simulink model "JT_60SA_scheme_japanese_sensors_isoflux_test_XSC"  (R2018a)
settings: Solver=ode45  StartTime=startTime-neg_time  StopTime=stopTime  FixedStep=5e-3  RelTol=1e-5
StartFcn:
  | coder.extrinsic('system');
  |  system('./run.csh')
  | 
  | 
  | 
  | disp('Called of the 1st part of the run.csh')
StopFcn:
  | close all
  | %figure
  | %run('../../JT-60SA simulation scheme/testPlot.m')
values from neighbouring files (symbols this model uses):
  A_contr = A    [JT60_CD_Invessel_simulator.m]    (also in JT_60SA_SOF18d66_japs_sensors_isoflux_simulator.m; JT_60SA_simulator_VS_SOF18d66_japs_sensors_isoflux_sqzd.m; getABCD (1).m = real(A_contr); getABCD.m = real(A_contr))
  B_contr = [B(:,[1:12 end]) A_contr*E]    [JT60_CD_Invessel_simulator.m]    (also in JT_60SA_SOF18d66_japs_sensors_isoflux_simulator.m; JT_60SA_simulator_VS_SOF18d66_japs_sensors_isoflux_sqzd.m; getABCD (1).m = [B_contr zeros(size(B_contr, 1), 2)]; getABCD.m = [B_contr, E([indexVD, indexEddy], :), Edot([indexVD, indexEd)
  C_contr = LinearModel.C(outputIdx,:)    [JT60_CD_Invessel_simulator.m]    (also in JT_60SA_SOF18d66_japs_sensors_isoflux_simulator.m; JT_60SA_simulator_VS_SOF18d66_japs_sensors_isoflux_sqzd.m; getABCD (1).m = [C1 C2] * T1; getABCD.m = [C1 C2] * T1)
  C_XSC_full = [C_PsiD; C_RxZx]    [XSC_isoflux_FBC.m]
  CSsat = [1 1.0 1.0 1] * 1e3    [JT60_CD_Invessel_simulator.m]    (also in JT_60SA_SOF18d66_japs_sensors_isoflux_simulator.m = [1 1.3 1.3 1] * 1e3; JT_60SA_simulator_VS_SOF18d66_japs_sensors_isoflux_sqzd.m = [1 1.3 1.3 1] * 1e3)
  D_contr = [LinearModel.D(outputIdx,[1:12 end]) LinearModel.F(outputIdx,:)+C_contr*E]    [JT60_CD_Invessel_simulator.m]    (also in JT_60SA_SOF18d66_japs_sensors_isoflux_simulator.m; JT_60SA_simulator_VS_SOF18d66_japs_sensors_isoflux_sqzd.m; getABCD (1).m = [D_contr zeros(size(C_contr, 1), 2)]; getABCD.m = [D_contr, D3])
  EFsat = [1 1.0 1.0 1.0 1.0 1] * 1e3    [JT60_CD_Invessel_simulator.m]    (also in JT_60SA_SOF18d66_japs_sensors_isoflux_simulator.m = [1 .97 .97 .97 .97 1] * 1e3; JT_60SA_simulator_VS_SOF18d66_japs_sensors_isoflux_sqzd.m = [1 .97 .97 .97 .97 1] * 1e3)
  equilDist = LinearModel.YEquil(LinearModel.DisturbancesInfo.OutputPosition)    [JT60_CD_Invessel_simulator.m]    (also in JT_60SA_SOF18d66_japs_sensors_isoflux_simulator.m; JT_60SA_simulator_VS_SOF18d66_japs_sensors_isoflux_sqzd.m)
  equilOutputs = LinearModel.YEquil(outputIdx)    [JT60_CD_Invessel_simulator.m]    (also in JT_60SA_SOF18d66_japs_sensors_isoflux_simulator.m; JT_60SA_simulator_VS_SOF18d66_japs_sensors_isoflux_sqzd.m)
  equilRxZx = LinearModel.YEquil(xIdx)    [JT60_CD_Invessel_simulator.m]    (also in JT_60SA_SOF18d66_japs_sensors_isoflux_simulator.m; JT_60SA_simulator_VS_SOF18d66_japs_sensors_isoflux_sqzd.m)
  equilVolts = zeros(11,1)    [JT60_CD_Invessel_simulator.m]    (also in JT_60SA_SOF18d66_japs_sensors_isoflux_simulator.m = zeros(13,1); JT_60SA_simulator_VS_SOF18d66_japs_sensors_isoflux_sqzd.m = zeros(13,1))
  eqXSC = [eqPsiCntr(2:end)-eqPsiX; eqRxZx]    [XSC_isoflux_FBC.m]
  I_sat_lower = [-3 -3 -3 -3 -3 -3 -3 -3 -3 -3]*1e4    [JT60_CD_Invessel_simulator.m]    (also in JT_60SA_SOF18d66_japs_sensors_isoflux_simulator.m = [-2 -2 -2 -2 -2 -2 -2 -2 -2 -2]*1e4; JT_60SA_simulator_VS_SOF18d66_japs_sensors_isoflux_sqzd.m = [-2 -2 -2 -2 -2 -2 -2 -2 -2 -2]*1e4)
  I_sat_upper = [3 3 3 3 3 3 3 3 3 3]*1e4    [JT60_CD_Invessel_simulator.m]    (also in JT_60SA_SOF18d66_japs_sensors_isoflux_simulator.m = [2 2 2 2 1 1 2 2 1 1]*1e4; JT_60SA_simulator_VS_SOF18d66_japs_sensors_isoflux_sqzd.m = [2 2 2 2 1 1 2 2 1 1]*1e4)
  kIp = kIp/norm(kIp)    [JT60_CD_Invessel_simulator.m]    (also in JT_60SA_SOF18d66_japs_sensors_isoflux_simulator.m; JT_60SA_simulator_VS_SOF18d66_japs_sensors_isoflux_sqzd.m)
  nOfFluxCntrl = nOfFluxCntrl +1    [JT60_CD_Invessel_simulator.m]    (also in JT_60SA_SOF18d66_japs_sensors_isoflux_simulator.m; JT_60SA_simulator_VS_SOF18d66_japs_sensors_isoflux_sqzd.m; MainConfigurator.m = 19)
  nOfFluxSens = 34    [JT60_CD_Invessel_simulator.m]    (also in JT_60SA_SOF18d66_japs_sensors_isoflux_simulator.m; JT_60SA_simulator_VS_SOF18d66_japs_sensors_isoflux_sqzd.m)
  nOfGaps = 85    [JT60_CD_Invessel_simulator.m]    (also in JT_60SA_SOF18d66_japs_sensors_isoflux_simulator.m; JT_60SA_simulator_VS_SOF18d66_japs_sensors_isoflux_sqzd.m)
  nOfMagneticSens = 45    [JT60_CD_Invessel_simulator.m]    (also in JT_60SA_SOF18d66_japs_sensors_isoflux_simulator.m; JT_60SA_simulator_VS_SOF18d66_japs_sensors_isoflux_sqzd.m)
  nOfStrikes = 8    [JT60_CD_Invessel_simulator.m]    (also in JT_60SA_SOF18d66_japs_sensors_isoflux_simulator.m; JT_60SA_simulator_VS_SOF18d66_japs_sensors_isoflux_sqzd.m)
  nXSC = size(C_XSC,1)    [XSC_isoflux_FBC.m]
  PSdelay = 1.5e-3    (= 0.0015)    [JT60_CD_Invessel_simulator.m]    (also in JT_60SA_SOF18d66_japs_sensors_isoflux_simulator.m; JT_60SA_simulator_VS_SOF18d66_japs_sensors_isoflux_sqzd.m)
  PSmodel = tf([1],[PStau 1]) * eye(nPF)    [JT60_CD_Invessel_simulator.m]    (also in JT_60SA_SOF18d66_japs_sensors_isoflux_simulator.m; JT_60SA_simulator_VS_SOF18d66_japs_sensors_isoflux_sqzd.m)
  r_cntrl_gap_eq = r_gap+initialGaps.*cosd(theta_cntrl_gap)    [JT60_CD_Invessel_simulator.m]    (also in JT_60SA_SOF18d66_japs_sensors_isoflux_simulator.m; JT_60SA_simulator_VS_SOF18d66_japs_sensors_isoflux_sqzd.m)
  vLoop = LinearModel.R(end,end)*Ip0    [JT60_CD_Invessel_simulator.m]    (also in JT_60SA_SOF18d66_japs_sensors_isoflux_simulator.m; JT_60SA_simulator_VS_SOF18d66_japs_sensors_isoflux_sqzd.m)
  xi0 = zeros(1, size(A_contr, 1))    [JT60_CD_Invessel_simulator.m]    (also in JT_60SA_SOF18d66_japs_sensors_isoflux_simulator.m; JT_60SA_simulator_VS_SOF18d66_japs_sensors_isoflux_sqzd.m)
  XSC_matrix = XSC_matrix(:, 1:end-1)    [XSC_3rd_try.m]    (also in XSC_SOF.mat = [-142.52465816 14.2057775457 0.338794355553 374.122305988 13; XSC_SOF_flux.mat = [-263113.154477 -155619.089697 161941.063761 -300901.385526 ; XSC_isoflux_FBC.m)
  z_cntrl_gap_eq = z_gap+initialGaps.*sind(theta_cntrl_gap)    [JT60_CD_Invessel_simulator.m]    (also in JT_60SA_SOF18d66_japs_sensors_isoflux_simulator.m; JT_60SA_simulator_VS_SOF18d66_japs_sensors_isoflux_sqzd.m)
undefined symbols (not defined in the file or in its folder): Input_struct, KPFcurr, VS
libraries: cstblocks x5, simulink x2
settings Model: Creator=Adriano  LastModifiedBy=dori
settings DataIOCC: LimitDataPoints=on  SaveFormat=Array
settings OptimizationCC: BlockReduction=off  BooleanDataType=off  LifeSpan=inf
settings DebuggingCC: SaveWithParameterizedLinksMsg=none  UnderspecifiedInitializationDetection=Classic  MergeDetectMultiDrivingBlocksExec=none  SignalResolutionControl=TryResolveAllWithWarning  AllowSymbolicDim=off  SFUnexpectedBacktrackingDiag=warning  SFNoUnconditionalDefaultTransitionDiag=warning  SFExecutionAtInitializationDiag=none
settings HardwareCC: ProdBitPerPointer=32  ProdBitPerSizeT=32  ProdBitPerPtrDiffT=32  ProdLargestAtomicFloat=None  ProdIntDivRoundTo=Undefined  ProdEndianess=Unspecified  ProdWordSize=32  ProdHWDeviceType=32-bit Generic  TargetUnknown=on
settings ModelReferenceCC: PropagateSignalLabelsOutOfModel=off
settings CodeAppCC: StateflowObjectComments=on
settings GRTTargetCC: TargetLangStandard=C89/C90 (ANSI)  GeneratePreprocessorConditionals=Disable all
settings ConfigComp: CovMetricSettings=dw  CovHtmlReporting=on  CovSaveCumulativeToWorkspaceVar=on  CovSaveSingleToWorkspaceVar=on  CovExternalEMLEnable=off

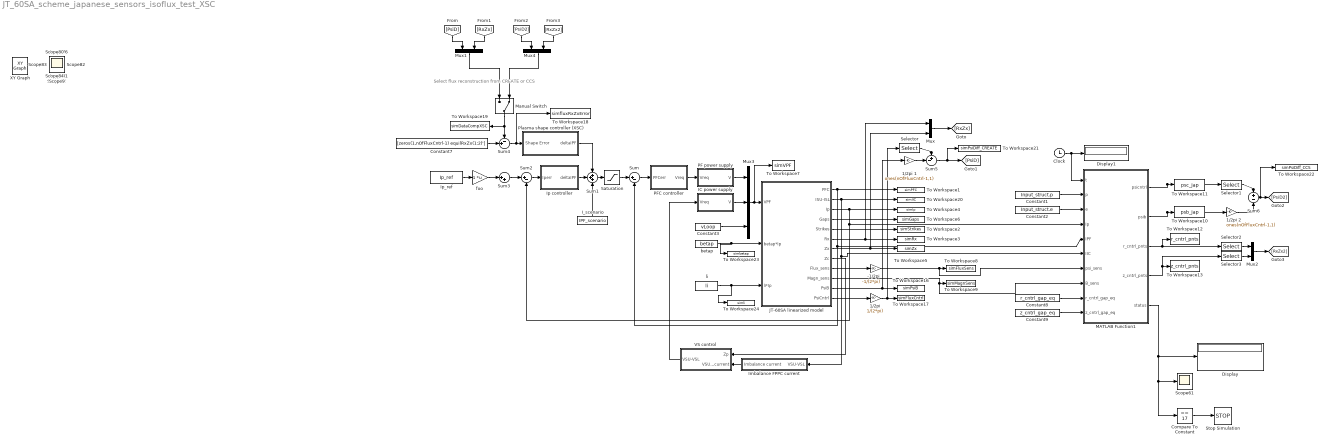
== system JT_60SA_scheme_japanese_sensors_isoflux_test_XSC ==
  note: Select flux reconstruction from CREATE or CCS
  -1/2pi : Gain  Gain=-1/(2*pi)
  "1/2pi " : Gain  Gain=1/(2*pi)
  1/2pi 1 : Gain  Gain=ones(nOfFluxCntrl-1,1)
  1/2pi 2 : Gain  Gain=ones(nOfFluxCntrl-1,1)
  Clock : Clock
  Compare To Constant : simulink/Logic and Bit Operations/Compare To Constant  relop===  const=17  OutDataTypeStr=boolean
  Constant1 : Constant  Value=Input_struct.p
  Constant2 : Constant  Value=Input_struct.e
  Constant3 : Constant  Value=vLoop
  Constant7 : Constant  Value=[zeros(1,nOfFluxCntrl-1) equilRxZx(1:2)']
  Constant8 : Constant  Value=r_cntrl_gap_eq
  Constant9 : Constant  Value=z_cntrl_gap_eq
  Display : Display
  Display1 : Display
  IC power supply : Subsystem
  I_scenario : FromWorkspace  VariableName=IPF_scenario  SampleTime=0  OutputAfterFinalValue=Holding final value
  Imbalance FPPC current : Subsystem
  Ip controller : Subsystem
  Ip_ref : FromWorkspace  VariableName=Ip_ref  SampleTime=0  OutputAfterFinalValue=Holding final value
  JT-60SA linearized model : Subsystem
  MATLAB Function1 : MATLAB Function  Description=CCS  StartFcn=|  TreatAsAtomicUnit=on  SystemSampleTime=25e-3
      | close all
      | figure(1)
  Manual Switch : ManualSwitch  CurrentSetting=0
  Mux : Mux  Inputs=2
  Mux1 : Mux  Inputs=[nOfFluxCntrl-1 2]
  Mux2 : Mux  Inputs=2
  Mux3 : Mux  Inputs=3
  Mux4 : Mux  Inputs=[nOfFluxCntrl-1 2]
  PF power supply : Subsystem
  PFC controller : Subsystem
  Plasma shape controller (XSC) : Subsystem
  Saturation : Saturate  UpperLimit=I_sat_upper  LowerLimit=I_sat_lower
  Scope{,1..84} (85 alike) : Scope
  Selector : Selector  InputPortWidth=nOfFluxCntrl  IndexOptions=Index vector (dialog)  Indices=[2:nOfFluxCntrl]  OutputSizes=1
  Selector1 : Selector  InputPortWidth=nOfFluxCntrl  IndexOptions=Index vector (dialog)  Indices=[2:nOfFluxCntrl]  OutputSizes=1
  Selector2 : Selector  InputPortWidth=nOfFluxCntrl  IndexOptions=Index vector (dialog)  Indices=1  OutputSizes=1
  Selector3 : Selector  InputPortWidth=nOfFluxCntrl  IndexOptions=Index vector (dialog)  Indices=1  OutputSizes=1
  Stop Simulation : Stop
  Sum : Sum  Inputs=|+-
  Sum1 : Sum  Inputs=+++
  Sum2 : Sum  Inputs=|+-
  Sum3 : Sum  Inputs=|++
  Sum4 : Sum  Inputs=-+|
  Sum5 : Sum  Inputs=+-|
  Sum6 : Sum  Inputs=+|-
  To Workspace1 : ToWorkspace  VariableName=simPFC  SaveFormat=Structure With Time  SampleTime=-1
  To Workspace10 : ToWorkspace  VariableName=psb_jap  SaveFormat=Structure With Time  SampleTime=-1
  To Workspace11 : ToWorkspace  VariableName=psc_jap  SaveFormat=Structure With Time  SampleTime=-1
  To Workspace12 : ToWorkspace  VariableName=r_cntrl_pnts  SaveFormat=Structure With Time  SampleTime=-1
  To Workspace13 : ToWorkspace  VariableName=z_cntrl_pnts  SaveFormat=Structure With Time  SampleTime=-1
  To Workspace16 : ToWorkspace  VariableName=simPsiB  SaveFormat=Structure With Time  SampleTime=-1
  To Workspace17 : ToWorkspace  VariableName=simFluxCntrl  SaveFormat=Structure With Time  SampleTime=-1
  To Workspace18 : ToWorkspace  VariableName=simfluxRxZxError  SaveFormat=Structure With Time  SampleTime=-1
  To Workspace19 : ToWorkspace  VariableName=simDataCompXSC  SaveFormat=Structure With Time  SampleTime=-1
  To Workspace2 : ToWorkspace  VariableName=simStrikes  SaveFormat=Structure With Time  SampleTime=-1
  To Workspace20 : ToWorkspace  VariableName=simIIC  SaveFormat=Structure With Time  SampleTime=-1
  To Workspace21 : ToWorkspace  VariableName=simPsiDiff_CREATE  SaveFormat=Structure With Time  SampleTime=-1
  To Workspace22 : ToWorkspace  VariableName=simPsiDiff_CCS  SaveFormat=Structure With Time  SampleTime=-1
  To Workspace23 : ToWorkspace  VariableName=simbetap  SaveFormat=Structure With Time  SampleTime=-1
  To Workspace24 : ToWorkspace  VariableName=simli  SaveFormat=Structure With Time  SampleTime=-1
  To Workspace3 : ToWorkspace  VariableName=simRx  SaveFormat=Structure With Time  SampleTime=-1
  To Workspace4 : ToWorkspace  VariableName=simIp  SaveFormat=Structure With Time  SampleTime=-1
  To Workspace5 : ToWorkspace  VariableName=simZx  SaveFormat=Structure With Time  SampleTime=-1
  To Workspace6 : ToWorkspace  VariableName=simGaps  SaveFormat=Structure With Time  SampleTime=-1
  To Workspace7 : ToWorkspace  VariableName=simVPF  SaveFormat=Structure With Time  SampleTime=-1
  To Workspace8 : ToWorkspace  VariableName=simFluxSens  SaveFormat=Structure With Time  SampleTime=-1
  To Workspace9 : ToWorkspace  VariableName=simMagnSens  SaveFormat=Structure With Time  SampleTime=-1
  VS control : Subsystem
  betap : FromWorkspace  VariableName=betap  SampleTime=0  OutputAfterFinalValue=Holding final value
  foo : Gain  Multiplication=Matrix(K*u)
  li : FromWorkspace  VariableName=li  SampleTime=0  OutputAfterFinalValue=Holding final value
  XY Graph : simulink/Sinks/XY Graph  IOType=viewer  xmin=-1  xmax=1  ymin=-1  ymax=1  st=-1
  wires:
  li/1 -> To Workspace24/1, JT-60SA linearized model/3(li*Ip)
  betap/1 -> To Workspace23/1, JT-60SA linearized model/2(betap*Ip)
  JT-60SA linearized model/1(PFC) -> MATLAB Function1/5(IPF), Sum/2, To Workspace1/1
  Mux3/1 -> To Workspace7/1, JT-60SA linearized model/1(VPF)
  Constant3/1 -> Mux3/3
  JT-60SA linearized model/3(Ip) -> Sum2/2, MATLAB Function1/4(Ip), To Workspace4/1
  JT-60SA linearized model/4(Gaps) -> To Workspace6/1
  JT-60SA linearized model/5(Strikes) -> To Workspace2/1
  JT-60SA linearized model/6(Rx) -> To Workspace3/1, Mux/1
  JT-60SA linearized model/7(Zx) -> To Workspace5/1, Mux/2
  Sum1/1 -> Saturation/1
  PF power supply/1(V) -> Mux3/1
  PFC controller/1(Vreq) -> PF power supply/1(Vreq)
  Sum2/1 -> Ip controller/1(Iperr)
  Sum3/1 -> Sum2/1
  Ip_ref/1 -> foo/1
  foo/1 -> Sum3/1
  Sum4/1 -> To Workspace18/1, Plasma shape controller (XSC)/1(Shape Error)
  Sum/1 -> PFC controller/1(PFCerr)
  Ip controller/1(deltaIPF) -> Sum1/2
  Saturation/1 -> Sum/1
  IC power supply/1(V) -> Mux3/2
  JT-60SA linearized model/8(Zc) -> VS control/1(Zp)
  JT-60SA linearized model/2(ISU-ISL) -> To Workspace20/1, Imbalance FPPC current/1(VSU-VSL), MATLAB Function1/6(IIC)
  Imbalance FPPC current/1(Imbalance current) -> VS control/2(VSU-VSL current)
  VS control/1(VSU-VSL) -> IC power supply/1(Vreq)
  I_scenario/1 -> Sum1/3
  MATLAB Function1/5(status) -> Compare To Constant/1, Scope61/1, Display/1
  Clock/1 -> MATLAB Function1/1(t), Display1/1
  Compare To Constant/1 -> Stop Simulation/1
  Constant1/1 -> MATLAB Function1/2(p)
  Constant2/1 -> MATLAB Function1/3(e)
  -1/2pi/1 -> To Workspace8/1, MATLAB Function1/7(psi_sens)
  JT-60SA linearized model/9(Flux_sens) -> -1/2pi/1
  JT-60SA linearized model/10(Magn_sens) -> To Workspace9/1, MATLAB Function1/8(B_sens)
  MATLAB Function1/1(psicntrl) -> Selector1/1, To Workspace11/1
  MATLAB Function1/2(psib) -> 1/2pi 2/1, To Workspace10/1
  MATLAB Function1/3(r_cntrl_pnts) -> To Workspace12/1, Selector2/1
  MATLAB Function1/4(z_cntrl_pnts) -> Selector3/1, To Workspace13/1
  Constant9/1 -> MATLAB Function1/10(z_cntrl_gap_eq)
  Constant8/1 -> MATLAB Function1/9(r_cntrl_gap_eq)
  JT-60SA linearized model/12(PsiCntrl) -> "1/2pi "/1
  JT-60SA linearized model/11(PsiB) -> 1/2pi 1/1, To Workspace16/1
  "1/2pi "/1 -> Selector/1, To Workspace17/1
  1/2pi 1/1 -> Sum5/2
  Mux/1 -> [RxZx]
  Sum5/1 -> To Workspace21/1, [PsiD]
  [PsiD] -> Mux1/1
  [RxZx] -> Mux1/2
  Constant7/1 -> Sum4/2
  Selector/1 -> Sum5/1
  Plasma shape controller (XSC)/1(deltaIPF) -> Sum1/1
  Selector1/1 -> Sum6/1
  1/2pi 2/1 -> Sum6/2
  Sum6/1 -> To Workspace22/1, [PsiD2]
  Mux2/1 -> [RxZx2]
  Selector2/1 -> Mux2/1
  Selector3/1 -> Mux2/2
  [PsiD2] -> Mux4/1
  [RxZx2] -> Mux4/2
  Manual Switch/1 -> To Workspace19/1, Sum4/1
  Mux1/1 -> Manual Switch/1
  Mux4/1 -> Manual Switch/2

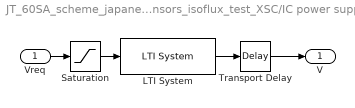
== system JT_60SA_scheme_japanese_sensors_isoflux_test_XSC/IC power supply ==
  Vreq : Inport
  LTI System : cstblocks/LTI System  sys=PSmodel(1:2, 1:2)  IC=[]
  Saturation : Saturate  UpperLimit=[1e3 1e3]  LowerLimit=[-1e3 -1e3]
  Transport Delay : TransportDelay  DelayTime=PSdelay
  V : Outport
  wires:
  LTI System/1 -> Transport Delay/1
  Vreq/1 -> Saturation/1
  Transport Delay/1 -> V/1
  Saturation/1 -> LTI System/1

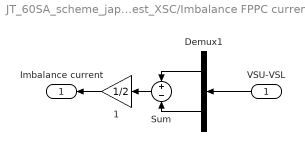
== system JT_60SA_scheme_japanese_sensors_isoflux_test_XSC/Imbalance FPPC current ==
  VSU-VSL : Inport
  "    1" : Gain  Gain=1/2
  Demux1 : Demux  Outputs=2
  Sum : Sum  Inputs=+|-
  Imbalance current : Outport
  wires:
  VSU-VSL/1 -> Demux1/1
  "    1"/1 -> Imbalance current/1
  Demux1/2 -> Sum/2
  Sum/1 -> "    1"/1
  Demux1/1 -> Sum/1

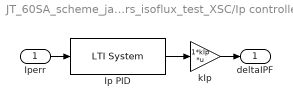
== system JT_60SA_scheme_japanese_sensors_isoflux_test_XSC/Ip controller ==
  Iperr : Inport
  Ip PID : cstblocks/LTI System  sys=Ip_PID  IC=[]
  kIp : Gain  Gain=1*kIp  Multiplication=Matrix(K*u)
  deltaIPF : Outport
  wires:
  Ip PID/1 -> kIp/1
  Iperr/1 -> Ip PID/1
  kIp/1 -> deltaIPF/1

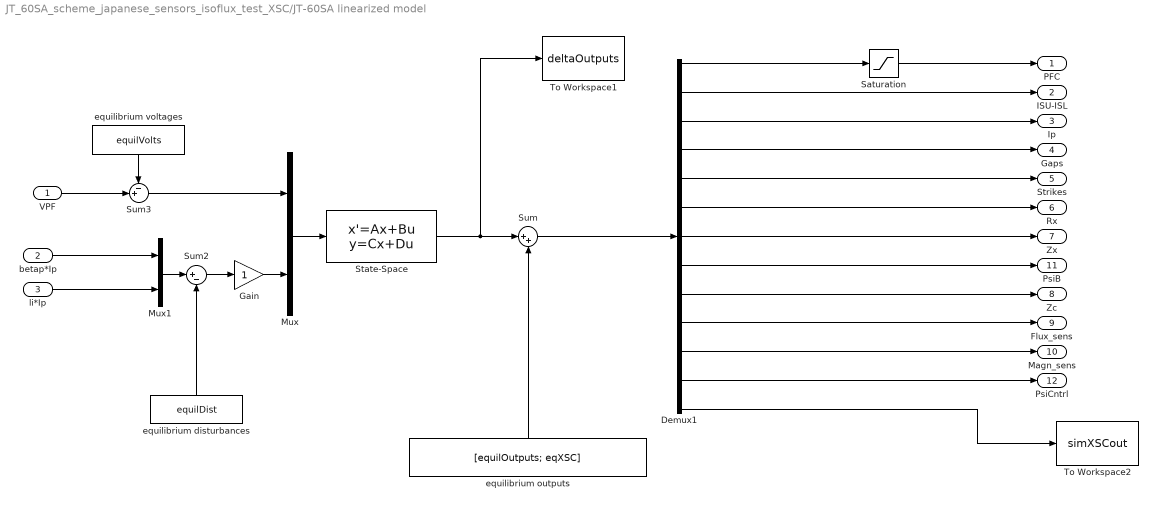
== system JT_60SA_scheme_japanese_sensors_isoflux_test_XSC/JT-60SA linearized model ==
  VPF : Inport
  betap*Ip : Inport  Port=2
  li*Ip : Inport  Port=3
  Demux1 : Demux  Outputs=[10 2 1 nOfGaps nOfStrikes 1 1 1 1 nOfFluxSens nOfMagneticSens nOfFluxCntrl nXSC]
  Gain : Gain
  Mux : Mux  Inputs=2
  Mux1 : Mux  Inputs=2
  Saturation : Saturate  UpperLimit=I_sat_upper  LowerLimit=I_sat_lower
  State-Space : StateSpace  A=A_contr  B=B_contr  C=[C_contr; C_XSC_full]  D=[D_contr; zeros(nXSC,size(D_contr,2))]  InitialCondition=xi0
  Sum : Sum  Inputs=|++
  Sum2 : Sum  Inputs=|+-
  Sum3 : Sum  Inputs=-+|
  To Workspace1 : ToWorkspace  VariableName=deltaOutputs  SaveFormat=Structure With Time  SampleTime=-1
  To Workspace2 : ToWorkspace  VariableName=simXSCout  SaveFormat=Structure With Time  SampleTime=-1
  equilibrium disturbances : Constant  Value=equilDist
  equilibrium outputs : Constant  Value=[equilOutputs; eqXSC]
  equilibrium voltages : Constant  Value=equilVolts
  PFC : Outport
  ISU-ISL : Outport  Port=2
  Ip : Outport  Port=3
  Gaps : Outport  Port=4
  Strikes : Outport  Port=5
  Rx : Outport  Port=6
  Zx : Outport  Port=7
  Zc : Outport  Port=8
  Flux_sens : Outport  Port=9
  Magn_sens : Outport  Port=10
  PsiB : Outport  Port=11
  PsiCntrl : Outport  Port=12
  wires:
  State-Space/1 -> To Workspace1/1, Sum/1
  Sum/1 -> Demux1/1
  equilibrium outputs/1 -> Sum/2
  Mux/1 -> State-Space/1
  VPF/1 -> Sum3/2
  Demux1/1 -> Saturation/1
  Mux1/1 -> Sum2/1
  equilibrium disturbances/1 -> Sum2/2
  betap*Ip/1 -> Mux1/1
  li*Ip/1 -> Mux1/2
  Sum3/1 -> Mux/1
  equilibrium voltages/1 -> Sum3/1
  Sum2/1 -> Gain/1
  Demux1/3 -> Ip/1
  Demux1/4 -> Gaps/1
  Demux1/5 -> Strikes/1
  Demux1/6 -> Rx/1
  Demux1/7 -> Zx/1
  Gain/1 -> Mux/2
  Saturation/1 -> PFC/1
  Demux1/2 -> ISU-ISL/1
  Demux1/9 -> Zc/1
  Demux1/11 -> Magn_sens/1
  Demux1/10 -> Flux_sens/1
  Demux1/8 -> PsiB/1
  Demux1/12 -> PsiCntrl/1
  Demux1/13 -> To Workspace2/1

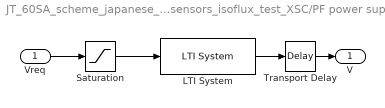
== system JT_60SA_scheme_japanese_sensors_isoflux_test_XSC/PF power supply ==
  Vreq : Inport
  LTI System : cstblocks/LTI System  sys=PSmodel  IC=[]
  Saturation : Saturate  UpperLimit=[CSsat EFsat]  LowerLimit=-[CSsat EFsat]
  Transport Delay : TransportDelay  DelayTime=PSdelay
  V : Outport
  wires:
  LTI System/1 -> Transport Delay/1
  Transport Delay/1 -> V/1
  Vreq/1 -> Saturation/1
  Saturation/1 -> LTI System/1

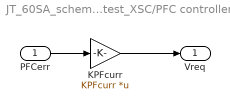
== system JT_60SA_scheme_japanese_sensors_isoflux_test_XSC/PFC controller ==
  PFCerr : Inport
  KPFcurr : Gain  Gain=KPFcurr  Multiplication=Matrix(K*u)
  Vreq : Outport
  wires:
  KPFcurr/1 -> Vreq/1
  PFCerr/1 -> KPFcurr/1

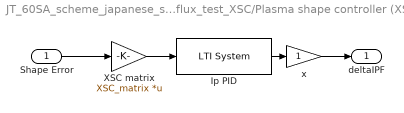
== system JT_60SA_scheme_japanese_sensors_isoflux_test_XSC/Plasma shape controller (XSC) ==
  Shape Error : Inport
  Ip PID : cstblocks/LTI System  sys=XSC_PI  IC=[]
  XSC matrix : Gain  Gain=XSC_matrix  Multiplication=Matrix(K*u)
  x : Gain
  deltaIPF : Outport
  wires:
  Shape Error/1 -> XSC matrix/1
  XSC matrix/1 -> Ip PID/1
  Ip PID/1 -> x/1
  x/1 -> deltaIPF/1

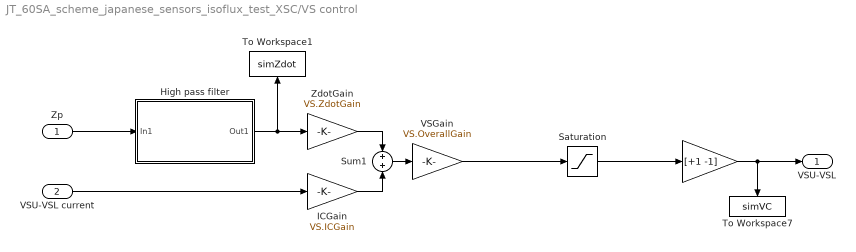
== system JT_60SA_scheme_japanese_sensors_isoflux_test_XSC/VS control ==
  Zp : Inport
  VSU-VSL current : Inport  Port=2
  "    " : Gain  Gain=[+1 -1]
  High pass filter : Subsystem
  ICGain : Gain  Gain=VS.ICGain
  Saturation : Saturate  UpperLimit=1e3  LowerLimit=-1e3
  Sum1 : Sum  Inputs=+|+
  To Workspace1 : ToWorkspace  VariableName=simZdot  SaveFormat=Structure With Time  SampleTime=-1
  To Workspace7 : ToWorkspace  VariableName=simVC  SaveFormat=Structure With Time  SampleTime=-1
  VSGain : Gain  Gain=VS.OverallGain
  ZdotGain : Gain  Gain=VS.ZdotGain
  VSU-VSL : Outport
  wires:
  VSU-VSL current/1 -> ICGain/1
  High pass filter/1(Out1) -> To Workspace1/1, ZdotGain/1
  Zp/1 -> High pass filter/1(In1)
  Sum1/1 -> VSGain/1
  ZdotGain/1 -> Sum1/1
  ICGain/1 -> Sum1/2
  "    "/1 -> VSU-VSL/1, To Workspace7/1
  VSGain/1 -> Saturation/1
  Saturation/1 -> "    "/1

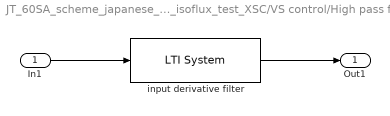
== system JT_60SA_scheme_japanese_sensors_isoflux_test_XSC/VS control/High pass filter ==
  In1 : Inport
  input derivative filter : cstblocks/LTI System  sys=VS.Filter  IC=[]
  Out1 : Outport
  wires:
  input derivative filter/1 -> Out1/1
  In1/1 -> input derivative filter/1

== matlab function JT_60SA_scheme_japanese_sensors_isoflux_test_XSC/MATLAB Function1 ==
  data: psicntrl output; psib output; r_cntrl_pnts output; z_cntrl_pnts output; t input; status output; p input; e input; Ip input; IPF input; IIC input; psi_sens input; B_sens input; r_cntrl_gap_eq input; z_cntrl_gap_eq input
 function [psicntrl,psib,r_cntrl_pnts,z_cntrl_pnts,status]= fcn(t,p,e,Ip,IPF,IIC,psi_sens,B_sens,r_cntrl_gap_eq,z_cntrl_gap_eq)

coder.extrinsic('system');
coder.extrinsic('run');
coder.extrinsic('num2str');
coder.extrinsic('pdemesh');
% coder.extrinsic('fscanf');
% coder.extrinsic('regexp');
% coder.extrinsic('int8');
% coder.extrinsic('fopen');


%%%%Fill the fort.70

%% Dummy data
% Ip = 5.5; %%is already in MA
Ip = Ip*1e-6;
IPF = IPF*1e-6;
IIC = IIC*1e-6;
%    psi_sens = psi_sens;
% IPF = [1 2 3 4 5 6 7 8 9 10]*1e3;
% IIC = [11 12]*1e3;
% B_sens = linspace(1e-1,5e-1,45); % 45 field sensors
% psi_sens = linspace(-0.5,2.5,34); % 34 flux loops


%%% Control points for isoflux
% ncp = length(r_cntrl_gap_eq);
% rcp = [0 1:10]; % 1st value must be zero?
% rcp=[0.00000000e+00, 4.00000000e+00, 3.60000000e+00, 2.10000000e+00 ,...
%     2.10000000e+00, 3.60000000e+00];

% zcp = [0 11:20];
% zcp=[ 0.00000000e+00, 0.00000000e+00, 1.10000000e+00,...
%     1.60000000e+00,-1.60000000e+00,-1.10000000e+00];

r_cntrl_gap_eq(1)=0;
rcp=r_cntrl_gap_eq';
z_cntrl_gap_eq(1)=0;
zcp=z_cntrl_gap_eq';
ncp = length(r_cntrl_gap_eq);


%%% Currents
% IPF=[-1.79500000e-03,-1.28500000e-02,-1.23900000e-02,...
%     -3.73900000e-03,-1.01300000e-02,-1.41700000e-02,...
%     1.36600000e-02, 1.02200000e-02, 3.63400000e-03,...
%     -1.87800000e-02];
% 
% IIC=[ 0.00000000e+00, 0.00000000e+00];
% 

%%% Field probes
% B_sens=[-2.93739000e-01, 1.64108000e-01, 1.31916100e+00, ...
%     1.87274400e+00, 2.08695600e+00, 2.16375900e+00, 2.09104000e+00,...
%     1.96193100e+00, 2.34451600e+00, 2.26190500e+00, 1.82612600e+00, ...
%     1.26108200e+00,-7.67500000e-02,-3.08937000e-01,-2.83100000e-03,...
%     2.02911000e-01, 3.29692000e-01, 3.53890000e-01, 3.11150000e-01,...
%     2.97641000e-01, 3.15344000e-01, 3.75148000e-01, 3.73400000e-01,...
%     3.05210000e-01,-6.57550000e-02,-4.77600000e-01,-4.74916000e-01,...
%     1.02603400e+00, 6.30836000e-01, 5.92683000e-01, 4.46055000e-01,...
%     6.33737000e-01, 6.58667000e-01, 5.40818000e-01];
% 

%%% Flux probes
% psi_sens=[5.76929000e-01, 6.72202000e-01, 6.65858000e-01, ...
%     6.35500000e-01, 6.52566000e-01, 6.74567000e-01, 5.16086000e-01, ...
%     1.81483000e-01,-3.24925000e-01,-3.84236000e-01,-9.20830000e-02,...
%     1.54298000e-01, 4.62897000e-01, 7.81376000e-01, 1.06759800e+00,...
%     1.12885400e+00, 1.05237800e+00, 7.74926000e-01, 4.94337000e-01,...
%     2.42900000e-01,-2.44260000e-02,-3.53074000e-01,-3.84375000e-01, ...
%     3.17130000e-02, 4.47325000e-01, 7.07756000e-01, 8.38931000e-01,...
%     7.53321000e-01, 6.39054000e-01, 5.45122000e-01, 5.94844000e-01,...
%     6.69196000e-01, 7.14051000e-01, 7.6384deg2rad+pi/23000e-01, 7.86789000e-01, ...
%     7.80176000e-01, 7.43075000e-01, 7.56568000e-01, 7.00523000e-01, ...
%     7.42489000e-01, 7.68867000e-01, 7.69857000e-01, 7.43815000e-01,...
%     7.00022000e-01, 6.19302000e-01];

%% Only if the time is bigger tahn some value
% if t > 0 && t< 0.5
if  1
    
matlab2namelist_smlnk2(t,Ip,IPF,IIC,B_sens,psi_sens,ncp,rcp,zcp);

%% Run ccs_sa
status=1;
status=system('./ccs_sa');

%% Select number of control points +1
cntrl_pnts= length(r_cntrl_gap_eq);

%% Extract control flux from fort.71
psib = 0;
psicntrl = zeros(cntrl_pnts,1);
 r_cntrl_pnts=zeros(cntrl_pnts,1);
 z_cntrl_pnts=zeros(cntrl_pnts,1);


[psib,psicntrl_all,r_cntrl_pnts_all,z_cntrl_pnts_all]=getFluxfort71();

psicntrl = psicntrl_all(1:cntrl_pnts,1);
 r_cntrl_pnts=r_cntrl_pnts_all(1:cntrl_pnts,1);
 z_cntrl_pnts=z_cntrl_pnts_all(1:cntrl_pnts,1);
% 
%% plot
figure(1)
run('./m1.m')
axis equal
xlim([0 5]);
title(['Time = ' num2str(t) 's'])
hold on
h = pdemesh(p,e,[]);
set(h, 'Color', 'k');
hold on
plot(rcp,zcp,'sr')
plot(r_cntrl_pnts, z_cntrl_pnts, 'g+')
hold off




 system('./run2.csh')



else
 status=1;  
 psib = 0;
 psicntrl = zeros(cntrl_pnts,1);
 r_cntrl_pnts=zeros(cntrl_pnts,1);
  z_cntrl_pnts=zeros(cntrl_pnts,1);

end
